simulink model "ramp_respose"  (R2020b)
settings: Solver=VariableStepAuto  StartTime=0.0  StopTime=10.0  RelTol=1e-3
model workspace: external: MATLAB File C:\Users\deves\MATLAB\Projects\problem5\data5.m (data not in the file)
values from neighbouring files (symbols this model uses):
  C = 10    [data5.m]
  R = 10    [data5.m]
libraries: simulink x1
settings Model: Creator=deves  LastModifiedBy=deves

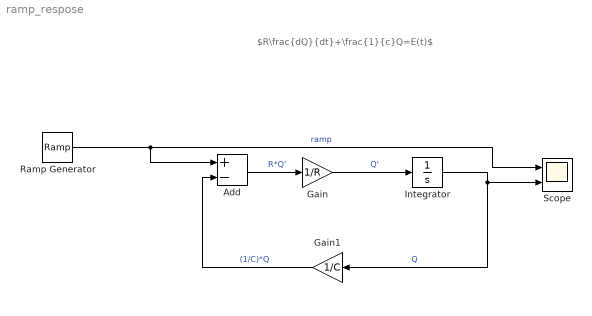
== system ramp_respose ==
  note: $R\frac{dQ}{dt}+\frac{1}{c}Q=E(t)$
  Add : Sum  Inputs=+-
  Gain : Gain  Gain=1/R
  Gain1 : Gain  Gain=1/C
  Integrator : Integrator  InitialCondition=5
  Ramp Generator : simulink/Sources/Ramp  slope=1  start=0  InitialOutput=0
  Scope : Scope  NumInputPorts=2
  wires:
  Integrator/1 -> Gain1/1, Scope/2  "Q"
  Ramp Generator/1 -> Scope/1, Add/1  "ramp"
  Gain/1 -> Integrator/1  "Q'"
  Gain1/1 -> Add/2  "(1/C)*Q"
  Add/1 -> Gain/1  "R*Q'"
